simulink model "solarModelClean"  (Simulink 10.1)
settings: Solver=VariableStepAuto  StartTime=0.0  StopTime=10.0  RelTol=1e-3
values from neighbouring files (symbols this model uses):
  opt = 75    [pr.mat]    (also in solor_irra_var.m = 30; solor_temp_var.m = temp(i))
  srad = 500    [pr.mat]    (also in solor_irra_var.m = srd(i); solor_temp_var.m)
libraries: simulink x2, powerlib x1
settings Model: Creator=shrad  LastModifiedBy=shrad
settings DataIOCC: SaveFormat=Dataset  ReturnWorkspaceOutputs=on
settings OptimizationCC: LifeSpan=auto
settings DebuggingCC: UnderspecifiedInitializationDetection=Simplified  MergeDetectMultiDrivingBlocksExec=error  SFUnexpectedBacktrackingDiag=error  SFNoUnconditionalDefaultTransitionDiag=error  SFExecutionAtInitializationDiag=warning  ArithmeticOperatorsInVariantConditions=error
settings HardwareCC: ProdBitPerPointer=64  ProdBitPerSizeT=64  ProdBitPerPtrDiffT=64  ProdLargestAtomicFloat=Float  ProdIntDivRoundTo=Zero  ProdEndianess=LittleEndian  ProdWordSize=64  ProdHWDeviceType=Intel->x86-64 (Windows64)
settings ModelReferenceCC: PropagateSignalLabelsOutOfModel=on
settings SFSimCC: SimUseLocalCustomCode=on  CustomCodeUndefinedFunction=FilterOut
settings RTWCC: RTWUseLocalCustomCode=on
settings CodeAppCC: StateflowObjectComments=off
settings GRTTargetCC: TargetLangStandard=C99 (ISO)  CombineOutputUpdateFcns=on  GRTInterface=off
settings ConfigComp: CovMetricSettings=dwe  CovHtmlReporting=off  CovSaveCumulativeToWorkspaceVar=off  CovSaveSingleToWorkspaceVar=off  CovExternalEMLEnable=on

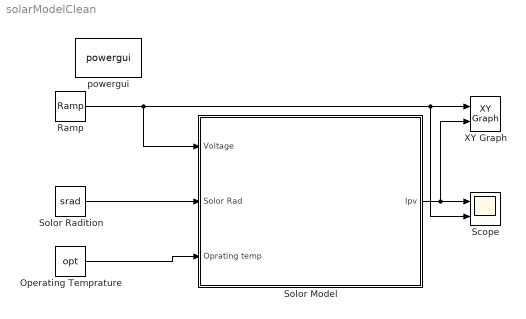
== system solarModelClean ==
  Operating Temprature : Constant  Value=opt
  Ramp : simulink/Sources/Ramp  slope=3  start=0  InitialOutput=0
  Scope : Scope  NumInputPorts=2
  Solor Model : Subsystem
  Solor Radition : Constant  Value=srad
  XY Graph : simulink/Sinks/XY Graph  xmin=-1  xmax=22  ymin=-1  ymax=10  st=-1
  powergui : powerlib/powergui  Priority=1  SimulationMode=Discrete  SampleTime=1e-6  frequency=60  Iterations=50  frequencyindice=0  Pbase=100e6  ErrMax=1e-4  UnitsV=kV  UnitsW=MW  buscounter=0  FunctionMessages=off  echomessages=off  EnableUseOfTLC=off  CurrentSourceSwitches=off  DisableSnubberDevices=off  DisableRonSwitches=off  DisableVfSwitches=off  DisplayEquations=off  AutomaticDiscreteSolvers=off  SolverType=Tustin  Interpol=off  ExternalGateDelay=off  methode=off  Ts=0  x0status=blocks  SPID=off  SwTol=0  HookPort=off  NonlinearTolerance=1e-4  nMaxIteration=100  ContinueOnMaxIteration=off  RestoreLinks=warning  ResistiveCurrentMeasurement=off  Frange=[0:2:500]  Ylog=off  Xlog=on  ShowGrid=off  save=off  variable=ZData  structure=0  ZoomFFT=off  StartTime=0.0  cycles=1  DisplayStyle=1  fundamental=60  FreqAxis=off  MaxFrequency=1000  frequencyindicesteady=1  RmsSteady=1  display=off
  wires:
  Solor Radition/1 -> Solor Model/2(Solor Rad)
  Operating Temprature/1 -> Solor Model/3(Oprating temp)
  Solor Model/1(Ipv) -> Scope/1, XY Graph/2
  Ramp/1 -> Scope/2, XY Graph/1, Solor Model/1(Voltage)

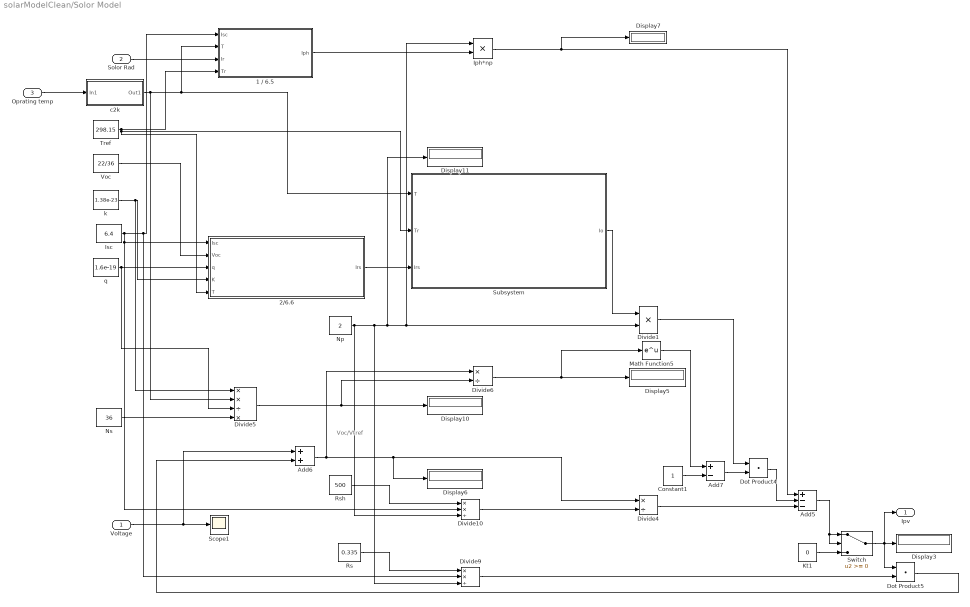
== system solarModelClean/Solor Model ==
  note: Voc/Vtref
  Voltage : Inport
  Solor Rad : Inport  Port=2
  Oprating temp : Inport  Port=3
  1 / 6.5 : Subsystem
  2/6.6 : Subsystem
  Add5 : Sum  Inputs=+--
  Add6 : Sum
  Add7 : Sum  Inputs=+-
  Constant1 : Constant
  Display{3,5..7,10..11} (6 alike) : Display
  Divide1 : Product
  Divide10 : Product  Inputs=**/
  Divide4 : Product  Inputs=*/
  Divide5 : Product  Inputs=**/*
  Divide6 : Product  Inputs=*/
  Divide9 : Product  Inputs=**/
  Dot Product4 : DotProduct  InputSameDT=on  OutDataTypeStr=Inherit: Inherit via internal rule
  Dot Product5 : DotProduct  InputSameDT=on  OutDataTypeStr=Inherit: Inherit via internal rule
  Iph*np : Product
  Isc : Constant  Value=6.4
  Kt1 : Constant  Value=0
  Math Function5 : Math  SignedPower=on  SaturateOnIntegerOverflow=on
  Np : Constant  Value=2
  Ns : Constant  Value=36
  Rs : Constant  Value=0.335
  Rsh : Constant  Value=500
  Scope1 : Scope
  Subsystem : Subsystem
  Switch : Switch
  Tref : Constant  Value=298.15
  Voc : Constant  Value=22/36
  c2k : Subsystem
  k : Constant  Value=1.38e-23
  q : Constant  Value=1.6e-19
  Ipv : Outport
  wires:
  Divide1/1 -> Dot Product4/1
  Voltage/1 -> Add6/1, Scope1/1
  Subsystem/1(Io) -> Divide1/1
  Divide10/1 -> Divide4/2
  Kt1/1 -> Switch/3
  Solor Rad/1 -> 1 / 6.5/3(Ir)
  1 / 6.5/1(Iph) -> Iph*np/2
  2/6.6/1(Irs) -> Subsystem/3(Irs)
  Voc/1 -> 2/6.6/2(Voc)
  Oprating temp/1 -> c2k/1(In1)
  Rsh/1 -> Divide10/1
  Divide9/1 -> Dot Product5/2
  Tref/1 -> 2/6.6/5(T), Subsystem/2(Tr), 1 / 6.5/4(Tr)
  Ns/1 -> Divide5/4
  Rs/1 -> Divide9/1
  Divide5/1 -> Display10/1, Divide6/2
  Math Function5/1 -> Add7/1
  Dot Product5/1 -> Add6/2
  Add7/1 -> Dot Product4/2
  Dot Product4/1 -> Add5/2
  Divide4/1 -> Add5/3
  Constant1/1 -> Add7/2
  k/1 -> Divide5/1, 2/6.6/4(K)
  Iph*np/1 -> Add5/1, Display7/1
  c2k/1(Out1) -> 1 / 6.5/2(T), Subsystem/1(T), Divide5/2
  Switch/1 -> Dot Product5/1, Ipv/1, Display3/1
  Np/1 -> Iph*np/1, Divide1/2, Display11/1, Divide9/3, Divide10/3
  Add5/1 -> Switch/2, Switch/1
  Divide6/1 -> Math Function5/1, Display5/1
  q/1 -> Divide5/3, 2/6.6/3(q)
  Add6/1 -> Divide4/1, Display6/1, Divide6/1
  Isc/1 -> 2/6.6/1(Isc), Divide10/2, 1 / 6.5/1(Isc), Divide9/2

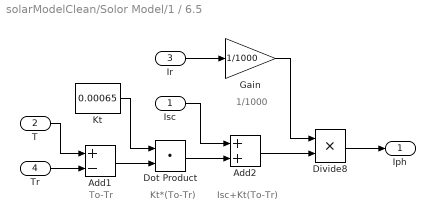
== system solarModelClean/Solor Model/1 / 6.5 ==
  note: To-Tr
  note: Kt*(To-Tr)
  note: Isc+Kt(To-Tr)
  note: 1/1000
  Isc : Inport
  T : Inport  Port=2
  Ir : Inport  Port=3
  Tr : Inport  Port=4
  Add1 : Sum  Inputs=+-
  Add2 : Sum
  Divide8 : Product
  Dot Product : DotProduct  InputSameDT=on  OutDataTypeStr=Inherit: Inherit via internal rule
  Gain : Gain  Gain=1/1000
  Kt : Constant  Value=0.00065
  Iph : Outport
  wires:
  Dot Product/1 -> Add2/2
  Kt/1 -> Dot Product/1
  Gain/1 -> Divide8/1
  Add1/1 -> Dot Product/2
  Add2/1 -> Divide8/2
  Tr/1 -> Add1/2
  Ir/1 -> Gain/1
  Isc/1 -> Add2/1
  T/1 -> Add1/1
  Divide8/1 -> Iph/1

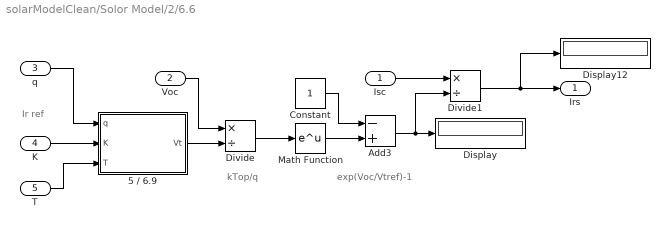
== system solarModelClean/Solor Model/2/6.6 ==
  note: kTop/q
  note: exp(Voc/Vtref)-1
  note: Ir ref
  Isc : Inport
  Voc : Inport  Port=2
  q : Inport  Port=3
  K : Inport  Port=4
  T : Inport  Port=5
  5 / 6.9 : Subsystem
  Add3 : Sum  Inputs=-+
  Constant : Constant
  Display : Display
  Display12 : Display
  Divide : Product  Inputs=*/
  Divide1 : Product  Inputs=*/
  Math Function : Math  SignedPower=on  SaturateOnIntegerOverflow=on
  Irs : Outport
  wires:
  q/1 -> 5 / 6.9/1(q)
  K/1 -> 5 / 6.9/2(K)
  T/1 -> 5 / 6.9/3(T)
  Constant/1 -> Add3/1
  Math Function/1 -> Add3/2
  Divide/1 -> Math Function/1
  5 / 6.9/1(Vt) -> Divide/2
  Isc/1 -> Divide1/1
  Divide1/1 -> Irs/1, Display12/1
  Voc/1 -> Divide/1
  Add3/1 -> Display/1, Divide1/2

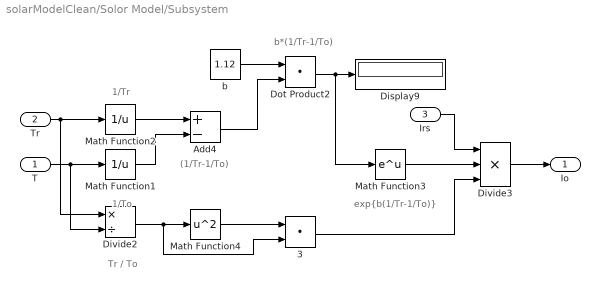
== system solarModelClean/Solor Model/Subsystem ==
  note: Tr / To
  note: 1/Tr
  note: 1/To
  note: (1/Tr-1/To)
  note: b*(1/Tr-1/To)
  note: exp{b(1/Tr-1/To)}
  T : Inport
  Tr : Inport  Port=2
  Irs : Inport  Port=3
  3 : DotProduct  InputSameDT=on  OutDataTypeStr=Inherit: Inherit via internal rule
  Add4 : Sum  Inputs=+-
  Display9 : Display
  Divide2 : Product  Inputs=*/
  Divide3 : Product  Inputs=3
  Dot Product2 : DotProduct  InputSameDT=on  OutDataTypeStr=Inherit: Inherit via internal rule
  Math Function1 : Math  Operator=reciprocal  SignedPower=on  SaturateOnIntegerOverflow=on
  Math Function2 : Math  Operator=reciprocal  SignedPower=on  SaturateOnIntegerOverflow=on
  Math Function3 : Math  SignedPower=on  SaturateOnIntegerOverflow=on
  Math Function4 : Math  Operator=square  SignedPower=on  SaturateOnIntegerOverflow=on
  b : Constant  Value=1.12
  Io : Outport
  wires:
  3/1 -> Divide3/3
  Divide3/1 -> Io/1
  Math Function2/1 -> Add4/1
  Math Function3/1 -> Divide3/2
  Math Function1/1 -> Add4/2
  Math Function4/1 -> 3/1
  Add4/1 -> Dot Product2/2
  Irs/1 -> Divide3/1
  b/1 -> Dot Product2/1
  T/1 -> Divide2/2, Math Function1/1
  Tr/1 -> Divide2/1, Math Function2/1
  Divide2/1 -> 3/2, Math Function4/1
  Dot Product2/1 -> Math Function3/1, Display9/1

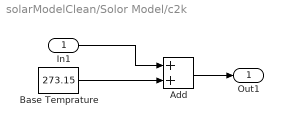
== system solarModelClean/Solor Model/c2k ==
  In1 : Inport
  Add : Sum
  Base Temprature : Constant  Value=273.15
  Out1 : Outport
  wires:
  Add/1 -> Out1/1
  Base Temprature/1 -> Add/2
  In1/1 -> Add/1

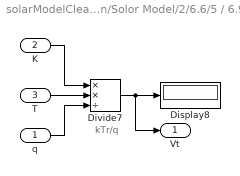
== system solarModelClean/Solor Model/2/6.6/5 / 6.9 ==
  note: kTr/q
  q : Inport
  K : Inport  Port=2
  T : Inport  Port=3
  Display8 : Display
  Divide7 : Product  Inputs=**/
  Vt : Outport
  wires:
  T/1 -> Divide7/2
  q/1 -> Divide7/3
  K/1 -> Divide7/1
  Divide7/1 -> Vt/1, Display8/1
